simulink model "linecodes"  (Simulink 7.9)
settings: Solver=VariableStepDiscrete  StartTime=0.0  StopTime=1  RelTol=1e-3
undefined symbols (not defined in the file): Rb, Spb
libraries: dspsigops x6, commutil2 x2, dspmathops x1
settings Model: Creator=mikael  LastModifiedBy=Marko  ExtModeAutoUpdateStatusClock=off
settings OptimizationCC: InitFltsAndDblsToZero=on
settings DebuggingCC: SaveWithParameterizedLinksMsg=none  FcnCallInpInsideContextMsg=Use local settings  StrictBusMsg=Warning
settings GRTTargetCC: TargetFcnLib=ansi_tfl_tmw.mat  CombineOutputUpdateFcns=off  GRTInterface=on

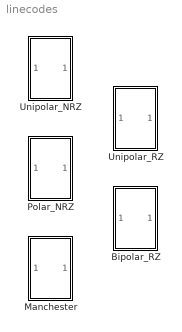
== system linecodes ==
  Bipolar_RZ : Subsystem  mask(Bipolar_rz){Rb=Rb, Spb=Spb}
      mask prompts: Rb "Binary Data Rate"; Spb "Sample per bit"
  Manchester : Subsystem  mask(Manchester){Rb=Rb, Spb=Spb}
      mask prompts: Rb "Binary Data Rate"; Spb "Samples per bit"
  Polar_NRZ : Subsystem  mask(Polar_nrz){Rb=Rb, Spb=Spb}
      mask prompts: Rb "Binary Data Rate"; Spb "Samples per bit"
  Unipolar_NRZ : Subsystem  mask(unipolar_nrz){Rb=Rb, Spb=Spb}
      mask prompts: Rb "Binary Data Rate"; Spb "Samples per bit"
  Unipolar_RZ : Subsystem  mask(Unipolar_rz){Rb=Rb, Spb=Spb}
      mask prompts: Rb "Binary Data Rate"; Spb "Samples per bit"

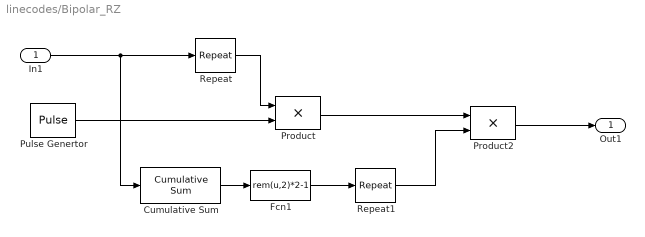
== system linecodes/Bipolar_RZ ==
  In1 : Inport
  Cumulative Sum : dspmathops/Cumulative Sum  dim=Channels (running sum)  reset_popup=None  roundingMode=Floor  overflowMode=off
  Fcn1 : Fcn  Expr=rem(u,2)*2-1
  Product : Product  SaturateOnIntegerOverflow=on  OutDataTypeStr=Inherit: Same as first input
  Product2 : Product  SaturateOnIntegerOverflow=on  OutDataTypeStr=Inherit: Same as first input
  Pulse Genertor : DiscretePulseGenerator  Period=Spb  PulseWidth=Spb/2  SampleTime=1/Rb/Spb  VectorParams1D=off
  Repeat : dspsigops/Repeat  N=Spb  ic=0  mode=Maintain input frame size
  Repeat1 : dspsigops/Repeat  N=Spb  ic=0  mode=Maintain input frame size
  Out1 : Outport
  wires:
  Repeat/1 -> Product/1
  Product2/1 -> Out1/1
  In1/1 -> Repeat/1, Cumulative Sum/1
  Fcn1/1 -> Repeat1/1
  Cumulative Sum/1 -> Fcn1/1
  Product/1 -> Product2/1
  Pulse Genertor/1 -> Product/2
  Repeat1/1 -> Product2/2

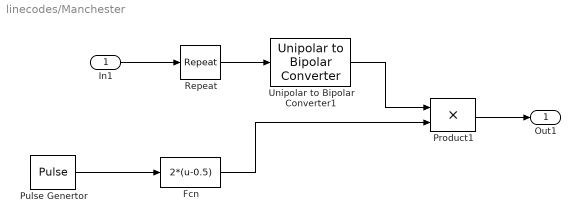
== system linecodes/Manchester ==
  In1 : Inport
  Fcn : Fcn  Expr=2*(u-0.5)
  Product1 : Product  SaturateOnIntegerOverflow=on  OutDataTypeStr=Inherit: Same as first input
  Pulse Genertor : DiscretePulseGenerator  Period=Spb  PulseWidth=Spb/2  SampleTime=1/Rb/Spb
  Repeat : dspsigops/Repeat  N=Spb  ic=0  mode=Maintain input frame size
  Unipolar to Bipolar Converter1 : commutil2/Unipolar to Bipolar Converter  SystemSampleTime=-1  M=2  polarity=Positive  dataType=Same as input
  Out1 : Outport
  wires:
  Product1/1 -> Out1/1
  In1/1 -> Repeat/1
  Pulse Genertor/1 -> Fcn/1
  Fcn/1 -> Product1/2
  Unipolar to Bipolar Converter1/1 -> Product1/1
  Repeat/1 -> Unipolar to Bipolar Converter1/1

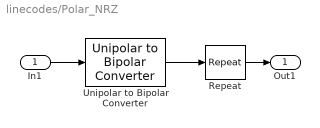
== system linecodes/Polar_NRZ ==
  In1 : Inport
  Repeat : dspsigops/Repeat  N=Spb  ic=0  mode=Maintain input frame size
  Unipolar to Bipolar Converter : commutil2/Unipolar to Bipolar Converter  SystemSampleTime=-1  M=2  polarity=Positive  dataType=Same as input
  Out1 : Outport
  wires:
  Unipolar to Bipolar Converter/1 -> Repeat/1
  In1/1 -> Unipolar to Bipolar Converter/1
  Repeat/1 -> Out1/1

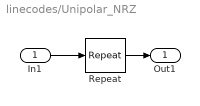
== system linecodes/Unipolar_NRZ ==
  In1 : Inport
  Repeat : dspsigops/Repeat  N=Spb  ic=0  mode=Maintain input frame size
  Out1 : Outport
  wires:
  In1/1 -> Repeat/1
  Repeat/1 -> Out1/1

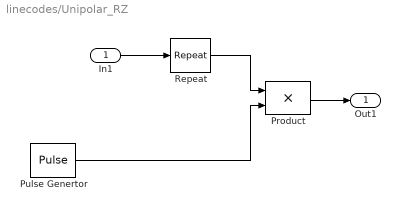
== system linecodes/Unipolar_RZ ==
  In1 : Inport
  Product : Product  SaturateOnIntegerOverflow=on  OutDataTypeStr=Inherit: Same as first input
  Pulse Genertor : DiscretePulseGenerator  Period=Spb  PulseWidth=Spb/2  SampleTime=1/Rb/Spb
  Repeat : dspsigops/Repeat  N=Spb  ic=0  mode=Maintain input frame size
  Out1 : Outport
  wires:
  In1/1 -> Repeat/1
  Pulse Genertor/1 -> Product/2
  Product/1 -> Out1/1
  Repeat/1 -> Product/1
